simulink model "Buck_converter_KF"  (R2020a)
settings: Solver=VariableStepAuto  StartTime=0.0  StopTime=4000  RelTol=1e-3
values from neighbouring files (symbols this model uses):
  A = [0 -1/L; -1/c 1/R*c]    [Kalman_filter_Params1.m]
  B = [1/L; 0]    [Kalman_filter_Params1.m]
  C = [1 0]    [Kalman_filter_Params1.m]
  c = 6.3    [Kalman_filter_Params1.m]    (also in UT.m = sqrt(c); myMeasurementFcn.m = 2.3; myStateTransitionFcn.m = 2.3)
  D = 0    [Kalman_filter_Params1.m]
  L = 3.23    [Kalman_filter_Params1.m]    (also in UT.m = size(X,2); myMeasurementFcn.m; myStateTransitionFcn.m)
  R = r*r    (= 0.04)    [EKF.m]    (also in KF.m = 4; Kalman_filter_Params1.m = 20; UKF_Test.m; myMeasurementFcn.m = 20)
  Vi = 10    [Kalman_filter_Params1.m]
  Vr = 4    [Kalman_filter_Params1.m]
undefined symbols (not defined in the file or in its folder): Continuous, Down, Time, Up
libraries: powerlib x8, ctrlSharedLib x1, eePwmGenerator x1
settings Model: Creator=NIKHIL  LastModifiedBy=NIKHIL
settings SolverCC: ZeroCrossAlgorithm=Adaptive
settings DebuggingCC: IgnoredZcDiagnostic=none

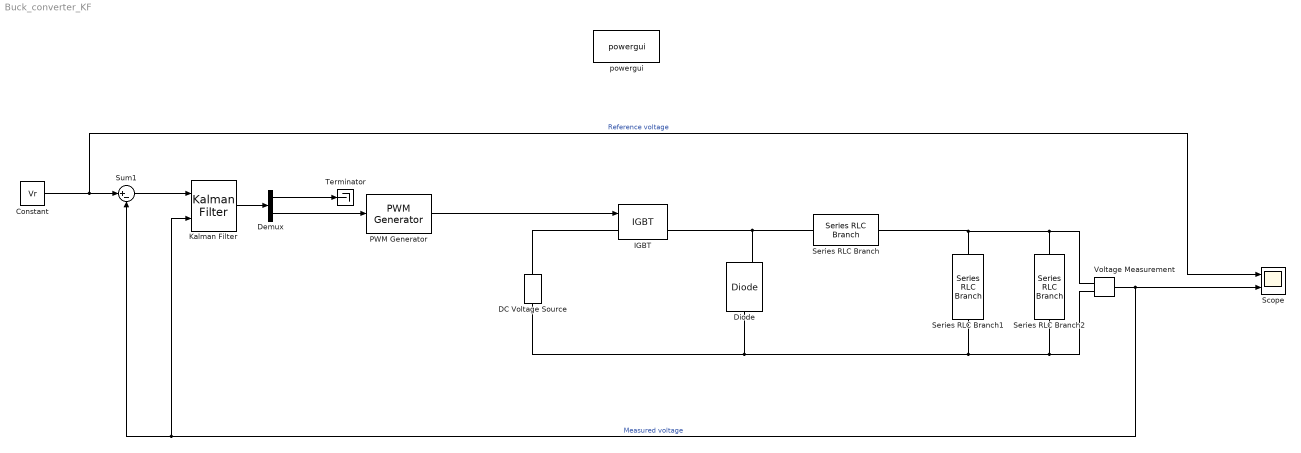
== system Buck_converter_KF ==
  Constant : Constant  Value=Vr
  DC Voltage Source : powerlib/Electrical Sources/DC Voltage Source  Amplitude=Vi  Measurements=None
  Demux : Demux  Outputs=2
  Diode : powerlib/Power Electronics/Diode  Ron=0.001  Lon=0  Vf=0.8  IC=0  UseSnubber=0  Rs=500  Cs=250e-9  Measurements=on
  IGBT : powerlib/Power Electronics/IGBT  Ron=0.001  Lon=0  Vf=1  Tf=1e-6  Tt=2e-6  IC=0  Rs=1e5  Cs=inf  Measurements=on
  Kalman Filter : ctrlSharedLib/Kalman Filter  TimeDomain=Continuous-Time  UseCurrentEstimator=on  ModelSource=Individual A, B, C, D matrices  ModelSourceVariable=ss(0.95,1,1,0,1)  A=A  B=B  C=C  D=D  NumberOfStates=1  NumberOfInputs=1  NumberOfOutputs=1  InitialEstimateSource=Dialog  X0=0  P0=10  UseK=off  UseGH=off  NumberOfProcessNoiseInputs=1  G=1  TimeInvariantG=on  H=0  TimeInvariantH=on  Q=0.05  TimeInvariantQ=on  R=1  TimeInvariantR=on  N=0  TimeInvariantN=on  AddInputPort=on  AddEnablePort=off  OutputEstimatedY=off  OutputP=off  Ts=5e-05
  PWM Generator : eePwmGenerator/PWM Generator  CarrCount=Up-Down  Tper=0.46  Ts=0
  Scope : Scope  NumInputPorts=2
  Series RLC Branch : powerlib/Elements/Series RLC Branch  LConnTagsString=__new0  RConnTagsString=__new0  BranchType=L  Resistance=1  Inductance=L  SetiL0=off  InitialCurrent=0  Capacitance=1e-6  Setx0=off  InitialVoltage=0  Measurements=None
  Series RLC Branch1 : powerlib/Elements/Series RLC Branch  LConnTagsString=__new0  RConnTagsString=__new0  BranchType=C  Resistance=1  Inductance=220e-3  SetiL0=off  InitialCurrent=0  Capacitance=c  Setx0=off  InitialVoltage=0  Measurements=None
  Series RLC Branch2 : powerlib/Elements/Series RLC Branch  LConnTagsString=__new0  RConnTagsString=__new0  BranchType=R  Resistance=R  Inductance=220e-3  SetiL0=off  InitialCurrent=0  Capacitance=220e-6  Setx0=off  InitialVoltage=0  Measurements=None
  Sum1 : Sum  Inputs=|+-
  Terminator : Terminator
  Voltage Measurement : powerlib/Measurements/Voltage Measurement  PhasorSimulation=off  OutputType=Complex  PSBequivalent=0
  powergui : powerlib/powergui  Priority=1  SimulationMode=Continuous  SampleTime=5e-05  frequency=60  Iterations=50  frequencyindice=0  Pbase=100e6  ErrMax=1e-4  UnitsV=kV  UnitsW=MW  buscounter=0  FunctionMessages=off  echomessages=off  EnableUseOfTLC=off  CurrentSourceSwitches=off  DisableSnubberDevices=off  DisableRonSwitches=off  DisableVfSwitches=off  DisplayEquations=off  AutomaticDiscreteSolvers=off  SolverType=Tustin/Backward Euler (TBE)  Interpol=off  ExternalGateDelay=off  methode=off  Ts=100  x0status=blocks  SPID=on  SwTol=0  HookPort=off  NonlinearTolerance=1e-4  nMaxIteration=100  ContinueOnMaxIteration=off  RestoreLinks=warning  ResistiveCurrentMeasurement=off  Frange=[0:2:500]  Ylog=off  Xlog=on  ShowGrid=off  save=off  variable=ZData  structure=0  ZoomFFT=off  StartTime=0.0  cycles=1  DisplayStyle=1  fundamental=60  FreqAxis=off  MaxFrequency=1000  frequencyindicesteady=1  RmsSteady=1  display=off
  wires:
  PWM Generator/1 -> IGBT/1
  Kalman Filter/1 -> Demux/1
  Voltage Measurement/1 -> Scope/2, Sum1/2, Kalman Filter/2  "Measured voltage"
  Constant/1 -> Sum1/1, Scope/1  "Reference voltage"
  Sum1/1 -> Kalman Filter/1
  Demux/2 -> PWM Generator/1
  Demux/1 -> Terminator/1
  connections:
  IGBT/LConn1 -- DC Voltage Source/RConn1
  IGBT/RConn1 -- Series RLC Branch/LConn1 -- Diode/RConn1
  DC Voltage Source/LConn1 -- Series RLC Branch2/RConn1 -- Voltage Measurement/LConn2 -- Series RLC Branch1/RConn1 -- Diode/LConn1
  Series RLC Branch1/LConn1 -- Voltage Measurement/LConn1 -- Series RLC Branch2/LConn1 -- Series RLC Branch/RConn1
